simulink model "untitled3"  (R2023b)
settings: Solver=VariableStepAuto  StartTime=0.0  StopTime=10.0  RelTol=1e-3
settings Model: Creator=A  LastModifiedBy=A

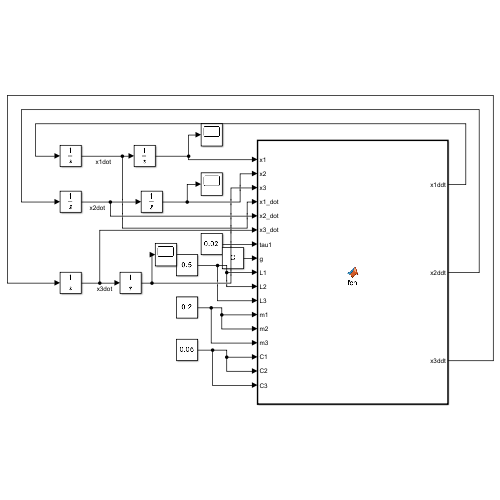
[thumbnail: Simulink's stored preview of the top-level diagram]
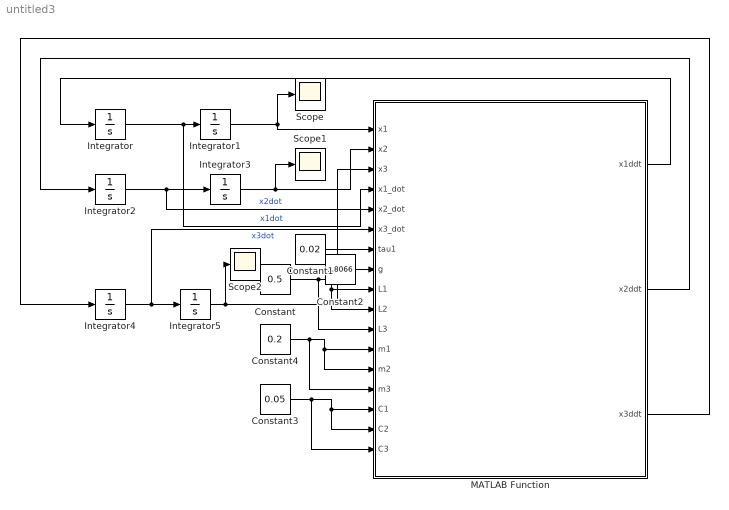
== system untitled3 ==
  Constant : Constant  Value=0.5
  Constant1 : Constant  Value=0.02
  Constant2 : Constant  Value=9.8066
  Constant3 : Constant  Value=0.05
  Constant4 : Constant  Value=0.2
  Integrator{,1..5} (6 alike) : Integrator
  MATLAB Function : MATLAB Function  TreatAsAtomicUnit=on
  Scope : Scope
  Scope1 : Scope
  Scope2 : Scope
  wires:
  Integrator/1 -> MATLAB Function/4(x1_dot), Integrator1/1  "x1dot"
  Integrator2/1 -> MATLAB Function/5(x2_dot), Integrator3/1  "x2dot"
  Integrator4/1 -> MATLAB Function/6(x3_dot), Integrator5/1  "x3dot"
  Integrator1/1 -> Scope/1, MATLAB Function/1(x1)
  Integrator3/1 -> Scope1/1, MATLAB Function/2(x2)
  Integrator5/1 -> Scope2/1, MATLAB Function/3(x3)
  MATLAB Function/1(x1ddt) -> Integrator/1
  MATLAB Function/2(x2ddt) -> Integrator2/1
  MATLAB Function/3(x3ddt) -> Integrator4/1
  Constant/1 -> MATLAB Function/11(L3), MATLAB Function/10(L2), MATLAB Function/9(L1)
  Constant1/1 -> MATLAB Function/7(tau1)
  Constant4/1 -> MATLAB Function/14(m3), MATLAB Function/13(m2), MATLAB Function/12(m1)
  Constant3/1 -> MATLAB Function/17(C3), MATLAB Function/16(C2), MATLAB Function/15(C1)
  Constant2/1 -> MATLAB Function/8(g)

== matlab function untitled3/MATLAB Function ==
  data: x1 input; x1ddt output; x2 input; x3 input; x1_dot input; x2_dot input; x3_dot input; tau1 input; g input; x2ddt output; x3ddt output; L1 input; L2 input; L3 input; m1 input; m2 input; m3 input; C1 input; C2 input; C3 input
function [x1ddt,x2ddt,x3ddt] = fcn(x1,x2,x3,x1_dot,x2_dot,x3_dot,tau1,g,L1,L2,L3,m1,m2,m3,C1,C2,C3)

I1=(m1/12)*L1*L1;
I2=(m2/12)*L2*L2;
I3=(m3/12)*L3*L3;

d11=I1 + I2/2 + I3/2 - (I3*cos(2*x2 + 2*x3))/2 + (L1^2*m1)/4 + L1^2*m2 + L1^2*m3 + (L2^2*m2)/8 + (L2^2*m3)/2 + (L3^2*m3)/8 - (I2*cos(2*x2))/2 - (L2^2*m2*cos(2*x2))/8 - (L2^2*m3*cos(2*x2))/2 - (L3^2*m3*cos(2*x2 + 2*x3))/8 + (L2*L3*m3*cos(x3))/2 - (L2*L3*m3*cos(2*x2 + x3))/2;
d12=-(L1*(L3*m3*cos(x2 + x3) + L2*m2*cos(x2) + 2*L2*m3*cos(x2)))/2;
d13=-(L1*L3*m3*cos(x2 + x3))/2;
d21=d12;
d22=I2 + I3 + (L2^2*m2)/4 + L2^2*m3 + (L3^2*m3)/4 + L2*L3*m3*cos(x3);
d23=(m3*L3^2)/4 + (L2*m3*cos(x3)*L3)/2 + I3;
d31=d13;
d32=d23;
d33=(m3*L3^2)/4 + I3;
Dq=[d11,d12,d13;
    d21,d22,d23;
    d31,d32,d33];


c11=I3*x1_dot*x2_dot*sin(2*x2 + 2*x3) + I3*x1_dot*x3_dot*sin(2*x2 + 2*x3) + I2*x1_dot*x2_dot*sin(2*x2) + (L1*L2*m2*x2_dot^2*sin(x2))/2 + L1*L2*m3*x2_dot^2*sin(x2) + (L2^2*m2*x1_dot*x2_dot*sin(2*x2))/4 + L2^2*m3*x1_dot*x2_dot*sin(2*x2) + (L3^2*m3*x1_dot*x2_dot*sin(2*x2 + 2*x3))/4 + (L3^2*m3*x1_dot*x3_dot*sin(2*x2 + 2*x3))/4 + (L1*L3*m3*x2_dot^2*sin(x2 + x3))/2 + (L1*L3*m3*x3_dot^2*sin(x2 + x3))/2 + L1*L3*m3*x2_dot*x3_dot*sin(x2 + x3) - (L2*L3*m3*x1_dot*x3_dot*sin(x3))/2 + L2*L3*m3*x1_dot*x2_dot*sin(2*x2 + x3) + (L2*L3*m3*x1_dot*x3_dot*sin(2*x2 + x3))/2;
c21= -(I3*x1_dot^2*sin(2*x2 + 2*x3))/2 - (I2*x1_dot^2*sin(2*x2))/2 - (L2^2*m2*x1_dot^2*sin(2*x2))/8 - (L2^2*m3*x1_dot^2*sin(2*x2))/2 - (L3^2*m3*x1_dot^2*sin(2*x2 + 2*x3))/8 - (L2*L3*m3*x3_dot^2*sin(x3))/2 - (L2*L3*m3*x1_dot^2*sin(2*x2 + x3))/2 - L2*L3*m3*x2_dot*x3_dot*sin(x3);
c31= ((L2*L3*m3*sin(x3))/4 - (L3^2*m3*sin(2*x2 + 2*x3))/8 - (I3*sin(2*x2 + 2*x3))/2 - (L2*L3*m3*sin(2*x2 + x3))/4)*x1_dot^2 + (L2*L3*m3*sin(x3)*x2_dot^2)/2;
cq=[c11;
    c21;
    c31];

g11=0;
g21=- g*m3*((L3*sin(x2 + x3))/2 + L2*sin(x2)) - (L2*g*m2*sin(x2))/2;
g31=-(L3*g*m3*sin(x2 + x3))/2;
Gq=[g11;
    g21;
    g31];

W11=C1*x1_dot;
W21=C2*x2_dot;
W31=C3*x3_dot;
Fi=[W11;
    W21;
    W31];

tau=[tau1;
    0;
    0];

ddx = Dq \ (tau - cq - Gq - Fi);
x1ddt=ddx(1,:);
x2ddt=ddx(2,:);
x3ddt=ddx(3,:);
